simulink model "may9js"  (R2015a)
settings: Solver=ode4  StartTime=0.0  StopTime=inf  FixedStep=BKIN_STEP_TIME  RelTol=1e-3
StartFcn:
  |  warndlg('Dexterit-E models cannot run under simulation. Please compile your model and run it from within Dexterit-E.');set_param(bdroot,'SimulationCommand','stop')
model workspace (MAT data in the model file):
  BARRIER_ROW = 5
  BKIN_KINEMATIC_FRAME_SIZE = 400
  BKIN_STEP_TIME = 0.00025
  CIRCLE_ROW = 2
  CIRCLE_STROKE = 10
  CIRCLE_STROKE_W = 11
  E_BARRIER_HIT = 6
  E_COLLISION_HIT = 7
  E_ENTER_PRESHOT_AREA = 2
  E_ENTER_START_AREA = 12
  E_EXIT = 13
  E_EXIT_PRESHOT_AREA = 10
  E_GOAL_HIT = 8
  E_GOAL_REACHED = 5
  E_NO_EVENT = 0
  E_PRESHOT_ROW = 4
  E_TARGET_OUT_OF_BOUNDS = 9
  E_TRIAL_BEGIN = 1
  E_TRIAL_ENDED = 3
  FIRST_STATE_FILL = 9
  FORCE_MULTIPLIER = 1
  F_BUMP = 1
  GOAL_ROW = 8
  GOAL_TIME = 15
  HEIGHT = 6
  INVISIBLE_FILL = 15
  LOAD_ROW = 4
  MASS_BARRIER = 6
  MASS_CIRCLE = 2
  MASS_RECT = 3
  NEW_FLOAT = 10
  NEW_ROW = 9
  NEW_TEXTSIZE = 11
  PERT_DUR = 5
  PERT_RAMP = 4
  PRESHOT_ROW = 7
  RADIUS_LOG = 4
  RADIUS_VIS = 5
  RECT_FILL = 12
  RECT_ROW = 3
  RECT_STROKE = 13
  RECT_STROKE_W = 14
  ROTATION = 7
  SECONDS = 1
  SECOND_STATE_FILL = 8
  SHOT_READY_TIME = 13
  SHOT_SET_TIME = 14
  START_HOLD_TIME = 12
  START_ROW = 6
  TRIAL_FAILURE = 11
  WIDTH = 3
  col_x = 1
  col_y = 2
undefined symbols (not defined in the file): slselsubs
libraries: Video x7, General x3, KINARM_loads x2, KINARM_EP_loads x1, KINARM_general x1, simulink x1, slrtlib x1
(part 4 of 4)

== matlab function may9js/PuckInTarget/Embedded MATLAB InsideTarget ==
  settings: fimath=|
      | fimath(...
      | 'RoundMode', 'floor',...
      | 'OverflowMode', 'wrap',...
      | 'ProductMode', 'KeepLSB', 'ProductWordLength', 32,...
      | 'SumMode', 'KeepLSB', 'SumWordLength', 32,...
      | 'CastBeforeSum', false)
  data: handpos input size=2; target_type input; attribcol input; num_targets input; intarget output; Target_Table input
function intarget = FIsInsideTarget(handpos, target_type, attribcol, num_targets, Target_Table)
% all dimensions in m, rad
% arguments:
% handpos: x,y positions of center of target
% attribcol: columns in target table specifying target attributes.  
% Specific to Target_Type
%	circle:
%	[X0,Y0,r...,rn] where:
%	X0,Y0 : centre of circle
%	r : logical radius of circle (i.e. radius used to determine 'in' or 'out' of target)
%	rn: logical radius of other targets (e.g. 2nd, 3rd) also specified in target row.
%   Up to 4 targets can be specified in a row
% ellipse:
%	[X0,Y0,a,b,t...,an, bn, tn] where:
%	X0,Y0 : centre of ellipse
%	a,b : major, minor radii of ellipse
%	t : rotation of ellipse in degrees
%	an,bn : major, minor radii of ellipse of other targets (e.g. 2nd, 3rd) also specified in target row
%	tn : rotation of ellipse in degrees of other targets (e.g. 2nd, 3rd) also specified in target row
%   Up to 4 targets can be specified in a row


target_col_x=1;
target_col_y=2;

x=handpos(1);
y=handpos(2);

intarget = zeros(size(Target_Table,1),5);

X0 = Target_Table(:,target_col_x)*0.01;			%Target Table sizes in cm in v1.4
Y0 = Target_Table(:,target_col_y)*0.01;			%Target Table sizes in cm in v1.4

deltax=x-X0;
deltay=y-Y0;

if target_type==1			%circle
	for target=1:num_targets
		r = Target_Table(:,attribcol(target))*0.01;			%Target Table sizes in cm in v1.4
		% simple euclidean distance
		distance2 = deltax.^2 + deltay.^2;					%distance2 is the square of the distance
	    intarget(:,target) = (distance2 <= r.^2);
	end
elseif target_type==2		%ellipse
	for target=1:num_targets
	    a = Target_Table(:,attribcol(target*3-2))*0.01;			%Target Table sizes in cm in v1.4
	    b = Target_Table(:,attribcol(target*3-1))*0.01;			%Target Table sizes in cm in v1.4	
	    t = Target_Table(:,attribcol(target*3))*(pi / 180.0);	%Target Table angles in degrees in v1.4
		sint=sin(t);
		cost=cos(t);
		xrotate=deltax.*cost+deltay.*sint;		%location of x point in ellipse's coordinate frame
		yrotate=-deltax.*sint+deltay.*cost;		%location of y point in ellipse's coordinate frame
		m=yrotate./xrotate;						%slope of line between the (x,y) to (x0,y0) in ellipse's coordinate frame
		y2sq=1./(1./(m.*a).^2+1./b.^2);			%y2sq is y2^2, where y2 is the intersection of the ellipse and the (x,y) to (x0,y0) line
	    intarget(:,target) = (yrotate.^2 <= y2sq);
    end
elseif target_type==3       %rectangle
    for target=1:num_targets
        w = Target_Table(:,attribcol(target*3-2))*0.01;  %width (sizes in cm in v1.4)
        h = Target_Table(:,attribcol(target*3-1))*0.01;  %height (sizes in cm in v1.4)
        
        if attribcol(target*3) > 0
            t = Target_Table(:,attribcol(target*3))*(pi / 180.0);  %angle (angles in degrees in v1.4)
        else
            t = zeros(size(Target_Table, 1), 1);
        end

        sint=sin(t);
        cost=cos(t);

        xrotate=deltax.*cost + deltay.*sint;   %location of x point in rectangle's coordinate frame
        yrotate=-deltax.*sint + deltay.*cost;  %location of y point in rectangle's coordinate frame

        intarget(:,target) = abs(xrotate) <= w/2 & abs(yrotate) <= h/2;
    end
elseif target_type==4       %line
    for target=1:num_targets
        % treat the line like a rectangle of height h and width w
        % determine height (stroke width) in the same fashion as in Show_Target
        if attribcol(target*3-2) == 0                     %0 column index means stroke width of 0
            h = zeros(size(Target_Table, 1), 1);
        elseif attribcol(target*3-2) < 0                  %-ve column index means stroke width of 1mm
            h = ones(size(Target_Table, 1), 1) .* 0.001;
        else
            h = Target_Table(:,attribcol(target*3-2)) * 0.01;  %target table contains width in cm
        end
        
        ex = Target_Table(:,attribcol(target*3-1))*0.01;  %endpoint in x relative to start point (cm)
        ey = Target_Table(:,attribcol(target*3))*0.01;    %endpoint in y relative to start point (cm)
        
        w = sqrt(ex.^2 + ey.^2);                          %width (cm)
        
        % determine the vector from the line's midpoint to the hand position
        handx = deltax - ex/2;
        handy = deltay - ey/2;
        
        t = atan2(ey, ex);                                %calculate angle of the line (rads)
        sint = sin(t);
        cost = cos(t);
        
        xrotate = handx.*cost + handy.*sint;   %location of x point in rectangle's coordinate frame
        yrotate = -handx.*sint + handy.*cost;  %location of y point in rectangle's coordinate frame
 
        intarget(:,target) = abs(xrotate) <= w/2 & abs(yrotate) <= h/2;
    end
elseif target_type==5  % triangle
    for target=1:num_targets
        w = Target_Table(:,attribcol(target*4-3))*0.01;         %length (sizes in cm in v1.4)
        
        % If a height column of 0 is specified, make the triangle equilateral. Otherwise, use the
        % values for height and peak offset from the target table.
        if attribcol(target*4-2) > 0
            h = Target_Table(:,attribcol(target*4-2))*0.01;  %height (sizes in cm in v1.4)
            p = Target_Table(:,attribcol(target*4-1))*0.01;  %peak offset (sizes in cm in v1.4)
        else
            h = w.*sin(pi/3.0);
            p = zeros(size(Target_Table, 1), 1);
        end
        
        if attribcol(target*4) > 0
            t = Target_Table(:,attribcol(target*4))*(pi / 180.0);  %angle (angles in degrees in v1.4)
        else
            t = zeros(size(Target_Table, 1), 1);
        end
        
        sint = sin(t);
        cost = cos(t);
        
        xrotate = deltax.*cost + deltay.*sint;   %location of x point in triangle's coordinate frame
        yrotate = -deltax.*sint + deltay.*cost;  %location of y point in triangle's coordinate frame
        
        % Perform a point-in-triangle test using Barycentric coordinates.
        A = [-w/2 - p/3, -h/3];
        B = [2*p/3, 2*h/3];
        C = [w/2 - p/3, -h/3];
        
        v0 = C - A;
        v1 = B - A;
        v2 = [xrotate, yrotate] - A;

        dot00 = v0(:,1) .* v0(:,1) + v0(:,2) .* v0(:,2);
        dot01 = v0(:,1) .* v1(:,1) + v0(:,2) .* v1(:,2);
        dot02 = v0(:,1) .* v2(:,1) + v0(:,2) .* v2(:,2);
        dot11 = v1(:,1) .* v1(:,1) + v1(:,2) .* v1(:,2);
        dot12 = v1(:,1) .* v2(:,1) + v1(:,2) .* v2(:,2);

        invDenom = 1 ./ (dot00 .* dot11 - dot01 .* dot01);
        u = (dot11 .* dot02 - dot01 .* dot12) .* invDenom;
        v = (dot00 .* dot12 - dot01 .* dot02) .* invDenom;

        intarget(:,target) = (u > 0) & (v > 0) & (u + v < 1);
    end
end

== matlab function may9js/Hand Feedback/Hand_Feedback/FeedFwdArm ==
  settings: fimath=|
      | fimath(...
      | 'RoundMode', 'floor',...
      | 'OverflowMode', 'wrap',...
      | 'ProductMode', 'KeepLSB', 'ProductWordLength', 32,...
      | 'SumMode', 'KeepLSB', 'SumWordLength', 32,...
      | 'CastBeforeSum', false)
  data: KINARMdata input; VCODES_in input; VCODES_out output; fdbk_stts_mdl input; block_settings input
function VCODES_out  = fcn(KINARMdata,VCODES_in,fdbk_stts_mdl, block_settings)
%
% This function creates the VCODEs for the hand position feedback for both
% hands.  Various options in the Mask of the Simulink block in which this
% embedded Matlab file sits, allow the user to specify how often
% the hand feedback is updated as well as the source of the style and status
% of the hand feedback.  
%
% block_settings is the value chosen by the user in the Mask for parent Simulink
% block.  Note: that even if the block is wired up to accept Task Program 
% control of hand feedback style and status, this embedded Matlab file allows
% the GUI to over-ride those settings.  However, if the GUI requests that
% the parent block use Task Program control for the style and/or status when
% it has not been programmed in, then this embedded Matlab file handles this
% appropriately and ignore the request for Task Program control.  
%
% block_settings=1 -- parent block does not have any Task Program control over style or status
% block_settings=2 -- parent block has Task Program control over status only
% block_settings=3 -- parent block has Task Program control over both style and status
%
% fdbk_stts_mdl (only potentially used if block_settings=2) 
% fdbk_stts_mdl=0 -- neither hand on
% fdbk_stts_mdl=1 -- dominant hand on
% fdbk_stts_mdl=2 -- non-dominant hand on
% fdbk_stts_mdl=3 -- both hands on
%
% VCODES (only potentially used if block_settings=3) 
% VCODES for dominant and non-dominant, input to parent block 


dominant_arm=KINARMdata(3,1);
feedfwd=KINARMdata(3,2);				%amount of feedforward extrapolation for hand position(s)
fdbk_stts_GUI=KINARMdata(3,3);			%status of hand feedback requested from GUI
fdbk_src_GUI=KINARMdata(3,4);			%source of hand feedback style requested from GUI
fdbk_clr_GUI=KINARMdata(3,5);			%colour of hand feedback required by GUI
fdbk_radius_GUI=KINARMdata(3,6);		%radius of hand feedback required by GUI


%----------------Feedback Style ----------------
% IF GUI asks for feedback style from Task Program (fdbk_src_GUI==0)
% AND if Task Program has been chosen to supply feedback style (block_settings==3)
% AND if Task Program actually supplies appropriate feedback styles (size(VCODES_in,2)==70)
if fdbk_src_GUI==0 && block_settings==3 && size(VCODES_in,2)==70
    VCODES=VCODES_in;
else
    VCODES=zeros(2,70);						%set default
	VCODES(:,1)=1;							%target_type of circle
	VCODES(:,5)=fdbk_clr_GUI;				%fill colour as specified by GUI
	VCODES(:,6)=fdbk_clr_GUI;				%stroke colour same as fill colour
	VCODES(:,7)=0;							%no stroke width
    VCODES(:,9)=100.0;                      %100% opacity
	VCODES(:,10)=fdbk_radius_GUI;			%radius (m) as specified by GUI
end

%----------------Feedback Status ----------------
%feedback status from GUI sets the default to be used
feedback_status=fdbk_stts_GUI;


if fdbk_stts_GUI==4				%if GUI has requested Task Program control of feedback status
	if block_settings==2		%if there is Task Program control ONLY of status (but not style)
		feedback_status=fdbk_stts_mdl;		%then use feedback status input from parent block
	elseif block_settings==3	%if there is Task Program control of both status and style
		feedback_status=4;		%then let the input VCODEs handle the status
	else						%otherwise assume that the Task Program did not provide style OR status
		feedback_status=3;		%then set both hands are always on as a default
    end
else		%if GUI is controlling feedback status
	feedback_status=fdbk_stts_GUI;
end

%set the status of the hand-feedback in the VCODES
switch feedback_status
	case 0					%show neither hand feedback
		VCODES(1,2)=0;
		VCODES(2,2)=0;
	case 1					%show ONLY dominant hand feedback
		VCODES(1,2)=1;
		VCODES(2,2)=0;
	case 2					%show ONLY non-dominant hand feedback
		VCODES(1,2)=0;
		VCODES(2,2)=1;
	case 4					%VCODES already control hand feedback
		%do nothing
	otherwise				%show both hand feedbacks
		VCODES(1,2)=1;
		VCODES(2,2)=1;
end

%----------------Feedback Position ----------------
%set the position of the hand feedback.
for i=1:2
	if i==1
		active_arm=KINARMdata(3,1);			%choose dominant arm first
	else
		active_arm=3-KINARMdata(3,1);		%choose non-dominant arm 2nd
	end
	HandXPos=KINARMdata(active_arm,23);		%(m)
	HandYPos=KINARMdata(active_arm,24);		%(m)
	HandXVel=KINARMdata(active_arm,25);		%(m/s)
	HandYVel=KINARMdata(active_arm,26);		%(m/s)

	% feed-forward hand position (m)
	%HandXPos_ff = HandXPos + HandXVel*feedfwd;
	%HandYPos_ff = HandYPos + HandYVel*feedfwd;
	HandXPos_ff = HandXPos;
	HandYPos_ff = HandYPos;
	VCODES(i,3)=HandXPos_ff;				%target position in m 
	VCODES(i,4)=HandYPos_ff;				%target position in m 
end

VCODES_out=VCODES;

== matlab function may9js/KINARM_HandInBarrier/Embedded MATLAB InsideTarget ==
  settings: fimath=|
      | fimath(...
      | 'RoundMode', 'floor',...
      | 'OverflowMode', 'wrap',...
      | 'ProductMode', 'KeepLSB', 'ProductWordLength', 32,...
      | 'SumMode', 'KeepLSB', 'SumWordLength', 32,...
      | 'CastBeforeSum', false)
  data: handpos input size=2; target_type input; attribcol input; num_targets input; intarget output; Target_Table input
function intarget = FIsInsideTarget(handpos, target_type, attribcol, num_targets, Target_Table)
% all dimensions in m, rad
% arguments:
% handpos: x,y positions of center of target
% attribcol: columns in target table specifying target attributes.  
% Specific to Target_Type
%	circle:
%	[X0,Y0,r...,rn] where:
%	X0,Y0 : centre of circle
%	r : logical radius of circle (i.e. radius used to determine 'in' or 'out' of target)
%	rn: logical radius of other targets (e.g. 2nd, 3rd) also specified in target row.
%   Up to 4 targets can be specified in a row
% ellipse:
%	[X0,Y0,a,b,t...,an, bn, tn] where:
%	X0,Y0 : centre of ellipse
%	a,b : major, minor radii of ellipse
%	t : rotation of ellipse in degrees
%	an,bn : major, minor radii of ellipse of other targets (e.g. 2nd, 3rd) also specified in target row
%	tn : rotation of ellipse in degrees of other targets (e.g. 2nd, 3rd) also specified in target row
%   Up to 4 targets can be specified in a row


target_col_x=1;
target_col_y=2;

x=handpos(1);
y=handpos(2);

intarget = zeros(size(Target_Table,1),5);

X0 = Target_Table(:,target_col_x)*0.01;			%Target Table sizes in cm in v1.4
Y0 = Target_Table(:,target_col_y)*0.01;			%Target Table sizes in cm in v1.4

deltax=x-X0;
deltay=y-Y0;

if target_type==1			%circle
	for target=1:num_targets
		r = Target_Table(:,attribcol(target))*0.01;			%Target Table sizes in cm in v1.4
		% simple euclidean distance
		distance2 = deltax.^2 + deltay.^2;					%distance2 is the square of the distance
	    intarget(:,target) = (distance2 <= r.^2);
	end
elseif target_type==2		%ellipse
	for target=1:num_targets
	    a = Target_Table(:,attribcol(target*3-2))*0.01;			%Target Table sizes in cm in v1.4
	    b = Target_Table(:,attribcol(target*3-1))*0.01;			%Target Table sizes in cm in v1.4	
	    t = Target_Table(:,attribcol(target*3))*(pi / 180.0);	%Target Table angles in degrees in v1.4
		sint=sin(t);
		cost=cos(t);
		xrotate=deltax.*cost+deltay.*sint;		%location of x point in ellipse's coordinate frame
		yrotate=-deltax.*sint+deltay.*cost;		%location of y point in ellipse's coordinate frame
		m=yrotate./xrotate;						%slope of line between the (x,y) to (x0,y0) in ellipse's coordinate frame
		y2sq=1./(1./(m.*a).^2+1./b.^2);			%y2sq is y2^2, where y2 is the intersection of the ellipse and the (x,y) to (x0,y0) line
	    intarget(:,target) = (yrotate.^2 <= y2sq);
    end
elseif target_type==3       %rectangle
    for target=1:num_targets
        w = Target_Table(:,attribcol(target*3-2))*0.01;  %width (sizes in cm in v1.4)
        h = Target_Table(:,attribcol(target*3-1))*0.01;  %height (sizes in cm in v1.4)
        
        if attribcol(target*3) > 0
            t = Target_Table(:,attribcol(target*3))*(pi / 180.0);  %angle (angles in degrees in v1.4)
        else
            t = zeros(size(Target_Table, 1), 1);
        end

        sint=sin(t);
        cost=cos(t);

        xrotate=deltax.*cost + deltay.*sint;   %location of x point in rectangle's coordinate frame
        yrotate=-deltax.*sint + deltay.*cost;  %location of y point in rectangle's coordinate frame

        intarget(:,target) = abs(xrotate) <= w/2 & abs(yrotate) <= h/2;
    end
elseif target_type==4       %line
    for target=1:num_targets
        % treat the line like a rectangle of height h and width w
        % determine height (stroke width) in the same fashion as in Show_Target
        if attribcol(target*3-2) == 0                     %0 column index means stroke width of 0
            h = zeros(size(Target_Table, 1), 1);
        elseif attribcol(target*3-2) < 0                  %-ve column index means stroke width of 1mm
            h = ones(size(Target_Table, 1), 1) .* 0.001;
        else
            h = Target_Table(:,attribcol(target*3-2)) * 0.01;  %target table contains width in cm
        end
        
        ex = Target_Table(:,attribcol(target*3-1))*0.01;  %endpoint in x relative to start point (cm)
        ey = Target_Table(:,attribcol(target*3))*0.01;    %endpoint in y relative to start point (cm)
        
        w = sqrt(ex.^2 + ey.^2);                          %width (cm)
        
        % determine the vector from the line's midpoint to the hand position
        handx = deltax - ex/2;
        handy = deltay - ey/2;
        
        t = atan2(ey, ex);                                %calculate angle of the line (rads)
        sint = sin(t);
        cost = cos(t);
        
        xrotate = handx.*cost + handy.*sint;   %location of x point in rectangle's coordinate frame
        yrotate = -handx.*sint + handy.*cost;  %location of y point in rectangle's coordinate frame
 
        intarget(:,target) = abs(xrotate) <= w/2 & abs(yrotate) <= h/2;
    end
elseif target_type==5  % triangle
    for target=1:num_targets
        w = Target_Table(:,attribcol(target*4-3))*0.01;         %length (sizes in cm in v1.4)
        
        % If a height column of 0 is specified, make the triangle equilateral. Otherwise, use the
        % values for height and peak offset from the target table.
        if attribcol(target*4-2) > 0
            h = Target_Table(:,attribcol(target*4-2))*0.01;  %height (sizes in cm in v1.4)
            p = Target_Table(:,attribcol(target*4-1))*0.01;  %peak offset (sizes in cm in v1.4)
        else
            h = w.*sin(pi/3.0);
            p = zeros(size(Target_Table, 1), 1);
        end
        
        if attribcol(target*4) > 0
            t = Target_Table(:,attribcol(target*4))*(pi / 180.0);  %angle (angles in degrees in v1.4)
        else
            t = zeros(size(Target_Table, 1), 1);
        end
        
        sint = sin(t);
        cost = cos(t);
        
        xrotate = deltax.*cost + deltay.*sint;   %location of x point in triangle's coordinate frame
        yrotate = -deltax.*sint + deltay.*cost;  %location of y point in triangle's coordinate frame
        
        % Perform a point-in-triangle test using Barycentric coordinates.
        A = [-w/2 - p/3, -h/3];
        B = [2*p/3, 2*h/3];
        C = [w/2 - p/3, -h/3];
        
        v0 = C - A;
        v1 = B - A;
        v2 = [xrotate, yrotate] - A;

        dot00 = v0(:,1) .* v0(:,1) + v0(:,2) .* v0(:,2);
        dot01 = v0(:,1) .* v1(:,1) + v0(:,2) .* v1(:,2);
        dot02 = v0(:,1) .* v2(:,1) + v0(:,2) .* v2(:,2);
        dot11 = v1(:,1) .* v1(:,1) + v1(:,2) .* v1(:,2);
        dot12 = v1(:,1) .* v2(:,1) + v1(:,2) .* v2(:,2);

        invDenom = 1 ./ (dot00 .* dot11 - dot01 .* dot01);
        u = (dot11 .* dot02 - dot01 .* dot12) .* invDenom;
        v = (dot00 .* dot12 - dot01 .* dot02) .* invDenom;

        intarget(:,target) = (u > 0) & (v > 0) & (u + v < 1);
    end
end

== stateflow chart may9js/Subsystem/Perturbation/Ramp_up_down ==
  state Perturbation/
    state on_ramp/
      entry: tick=0;
      on e_clk: tick++;
      scaling=tick/ramp_up;
    state peak/
      entry: scaling=1;
    state off_ramp
      entry: tick=0;
      scaling=1;
      on e_clk: tick++;
      scaling=1-tick/ramp_down;
    (junction 18) -> on_ramp [order 1] : [ramp_up > 0]
    (junction 18) -> (junction 20) [order 2]
    on_ramp -> (junction 20) : after(ramp_up, e_clk)
    (junction 20) -> peak [order 1] : [duration > 0]
    (junction 20) -> (junction 19) [order 2]
    peak -> (junction 19) : after(duration, e_clk)
    (junction 19) -> off_ramp [order 1] : [ramp_down > 0]
  state wait_for_trigger/
    entry: scaling=0;
  (default) -> wait_for_trigger
  wait_for_trigger -> (junction 18) : e_trigger
  Perturbation -> wait_for_trigger : e_reset
  (junction 19) -> wait_for_trigger [order 2]
  off_ramp -> wait_for_trigger : after(ramp_down, e_clk)
  data: ramp_up input double; duration input double; ramp_down input double; scaling output double; tick local double
  events: e_clk input RISING_EDGE_EVENT; e_trigger input EITHER_EDGE_EVENT; e_reset input EITHER_EDGE_EVENT

== matlab function may9js/Subsystem/Perturbation/Select Perturbation Times ==
  settings: fimath=|
      | fimath(...
      | 'RoundMode', 'floor',...
      | 'OverflowMode', 'wrap',...
      | 'ProductMode', 'KeepLSB', 'ProductWordLength', 32,...
      | 'SumMode', 'KeepLSB', 'SumWordLength', 32,...
      | 'CastBeforeSum', false)
  data: load_table input; load_row input; load_cols input; perturbation output
function perturbation  = select_times(load_table, load_row, load_cols)

% Select perturbation ramp up, duration, and ramp down times from the 
% from load table, or use 0 if an invalid load row and/or column is specified.

ramp_up = 0.0;
duration = 0.0;
ramp_down = 0.0;

if load_row > 0 && load_row <= size(load_table, 1)
    if load_cols(1) > 0
        ramp_up = load_table(load_row, load_cols(1));
    end
    if load_cols(2) > 0
        duration = load_table(load_row, load_cols(2));
    end
    if load_cols(3) > 0
        ramp_down = load_table(load_row, load_cols(3));
    end
end
        
perturbation = [ramp_up, duration, ramp_down];

== matlab function may9js/Hand Feedback/MATLAB Function ==
  data: feedback_vcodes input; arm_to_be_assessed input; hand_vcodes output
function hand_vcodes = fcn(feedback_vcodes, arm_to_be_assessed)
% the hand feedback vcodes are sorted like this:
%    <arm to be assessed vcode>
%    <contralateral arm> 
% but using this function I am going to sort the vcodes like this:
%    <right arm>
%    <left arm>
% because that will make it easier to track velocities and forces

if arm_to_be_assessed == 1
	hand_vcodes = feedback_vcodes;
else
	hand_vcodes = feedback_vcodes([2 1], :);
	%hand_vcodes = feedback_vcodes;
end
